simulink model "QuadrotorEulerModel"  (R2015b)
settings: Solver=VariableStepAuto  StartTime=0.0  StopTime=10.0  RelTol=1e-3
undefined symbols (not defined in the file): Initial
settings Model: Creator=jeremie  LastModifiedBy=jban039
settings ModelReferenceCC: ModelReferenceMinAlgLoopOccurrences=on

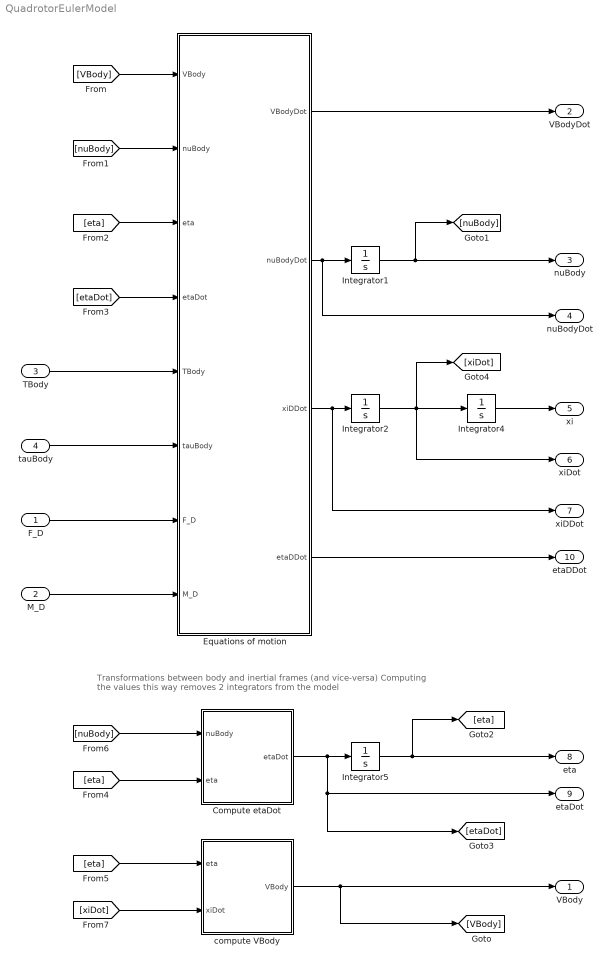
== system QuadrotorEulerModel ==
  note: Transformations between body and inertial frames (and vice-versa)
      | Computing the values this way removes 2 integrators from the model
  F_D : Inport
  M_D : Inport  Port=2
  TBody : Inport  Port=3
  tauBody : Inport  Port=4
  Compute etaDot : MATLAB Function  TreatAsAtomicUnit=on
  Equations of motion : MATLAB Function  TreatAsAtomicUnit=on
  Integrator1 : Integrator  InitialCondition=Initial.NU_BODY
  Integrator2 : Integrator  InitialCondition=Initial.XI_DOT
  Integrator4 : Integrator  InitialCondition=Initial.XI
  Integrator5 : Integrator  InitialCondition=Initial.ETA
  compute VBody : MATLAB Function  TreatAsAtomicUnit=on
  VBody : Outport
  VBodyDot : Outport  Port=2
  nuBody : Outport  Port=3
  nuBodyDot : Outport  Port=4
  xi : Outport  Port=5
  xiDot : Outport  Port=6
  xiDDot : Outport  Port=7
  eta : Outport  Port=8
  etaDot : Outport  Port=9
  etaDDot : Outport  Port=10
  wires:
  Equations of motion/1(VBodyDot) -> VBodyDot/1
  Integrator2/1 -> [xiDot], Integrator4/1, xiDot/1
  Integrator4/1 -> xi/1
  [nuBody] -> Equations of motion/2(nuBody)
  [VBody] -> Equations of motion/1(VBody)
  Integrator5/1 -> eta/1, [eta]
  [eta] -> Equations of motion/3(eta)
  [etaDot] -> Equations of motion/4(etaDot)
  tauBody/1 -> Equations of motion/6(tauBody)
  TBody/1 -> Equations of motion/5(TBody)
  Equations of motion/3(xiDDot) -> Integrator2/1, xiDDot/1
  Equations of motion/4(etaDDot) -> etaDDot/1
  F_D/1 -> Equations of motion/7(F_D)
  Compute etaDot/1(etaDot) -> Integrator5/1, [etaDot], etaDot/1
  [eta] -> Compute etaDot/2(eta)
  compute VBody/1(VBody) -> [VBody], VBody/1
  [eta] -> compute VBody/1(eta)
  M_D/1 -> Equations of motion/8(M_D)
  Integrator1/1 -> [nuBody], nuBody/1
  Equations of motion/2(nuBodyDot) -> nuBodyDot/1, Integrator1/1
  [nuBody] -> Compute etaDot/1(nuBody)
  [xiDot] -> compute VBody/2(xiDot)

== matlab function QuadrotorEulerModel/Equations of motion ==
  data: VBody input; VBodyDot output; nuBody input; eta input; etaDot input; TBody input size=3; tauBody input size=3; F_D input size=3; M_D input size=3; nuBodyDot output; Uav parameter; xiDDot output; etaDDot output
function [VBodyDot, nuBodyDot, xiDDot, etaDDot] = QuadrotorEulerModel(...
    VBody, nuBody, eta, etaDot, TBody, tauBody, F_D, M_D, Uav)
%#codegen

%% Rotation matrices
% Precompute sines and cosines
sPhi   = sin(eta(1));
sTheta = sin(eta(2));
sPsi   = sin(eta(3));
cPhi   = cos(eta(1));
cTheta = cos(eta(2));
cPsi   = cos(eta(3));
tTheta = tan(eta(2));

phiDot   = etaDot(1);
thetaDot = etaDot(2);

% Body frame to inertial frame
R = [cPsi*cTheta, cPsi*sTheta*sPhi-sPsi*cPhi, cPsi*sTheta*cPhi+sPsi*sPhi;
     sPsi*cTheta, sPsi*sTheta*sPhi+cPsi*cPhi, sPsi*sTheta*cPhi-cPsi*sPhi;
     -sTheta,     cTheta*sPhi,                cTheta*cPhi+sPsi*sPhi];

WInvertDot = [...
    0,  phiDot*cPhi*tTheta+thetaDot*sPhi/cTheta^2,    -phiDot*sPhi*cTheta+thetaDot*cPhi/cTheta^2;
    0, -phiDot*sPhi,                                  -phiDot*cPhi;
	0,  phiDot*cPhi/cTheta+phiDot*sPhi*tTheta/cTheta, -phiDot*sPhi/cTheta+thetaDot*cPhi*tTheta/cTheta];

WInvert = [1, sPhi*tTheta,  cPhi*tTheta;
           0, cPhi,        -sPhi;
           0, sPhi/cTheta,  cPhi/cTheta];

%% Moments and Forces
% Body frame accelerations
VBodyDot  = (1/Uav.M) * (R'*Uav.G + TBody - cross(nuBody, Uav.M*VBody) - F_D);
nuBodyDot = Uav.I \ (tauBody - cross(nuBody, Uav.I*nuBody) - M_D);

% Inertial frame accelerations
xiDDot = (1/Uav.M)*(Uav.G + R*TBody - R*F_D);
etaDDot = WInvertDot*nuBody + WInvert*nuBodyDot;

% Check centripetal force in inertial frame
% F_C = R*cross(nuBody,m*VBody);
end

== matlab function QuadrotorEulerModel/Compute etaDot ==
  data: nuBody input; eta input; etaDot output
function etaDot = computeEtaDot(nuBody, eta)
%#codegen

sPhi = sin(eta(1));
cPhi = cos(eta(1));
cTheta = cos(eta(2));
tTheta = tan(eta(2));
      
WInverse = [1, sPhi*tTheta,  cPhi*tTheta;
            0, cPhi,        -sPhi;
            0, sPhi/cTheta,  cPhi/cTheta];

etaDot = WInverse*nuBody;

== matlab function QuadrotorEulerModel/compute VBody ==
  data: eta input; VBody output; xiDot input
function VBody = computeVBody(eta, xiDot)
%#codegen

sphi = sin(eta(1));
sTheta = sin(eta(2));
sPsi = sin(eta(3));
cPhi = cos(eta(1));
cTheta = cos(eta(2));
cPsi = cos(eta(3));

R = [ cPsi*cTheta, cPsi*sTheta*sphi-sPsi*cPhi, cPsi*sTheta*cPhi+sPsi*sphi;
	  sPsi*cTheta, sPsi*sTheta*sphi+cPsi*cPhi, sPsi*sTheta*cPhi-cPsi*sphi;
     -sTheta,      cTheta*sphi,                cTheta*cPhi+sPsi*sphi];

VBody = R'*xiDot;
